simulink model "DFIG_BESS_In_power_LFnetwork_5bus"  (R2017b)
settings: Solver=ode23tb  StartTime=0.0  StopTime=7.5  MaxStep=0.04  RelTol=1e-3  EnableMultiTasking=on
undefined symbols (not defined in the file or in its folder): beta, Cbus, Cbus_bess, Cfilter, cp_opt_abs, D, D1, D11, Delta, DiscIntNeverNeededParam, f, Fs, fsw, Ion, J, ki_id, ki_idg, ki_iq, ki_iqg, ki_v, kp_id, kp_idg, kp_iq, kp_iqg, kp_v, Kpg, Kqg, lambda_opt, Lfilter, Lg, Lithium, Lm, Lr, Ls, Lsi, n, N, p, Ps, Radio, Rfilter, ro, Rr, Rs, sigbuilder_block, sigma, Ts, Vbus_ref, Vdc_bat_ref, Vs
libraries: powerlib x83, powerlib_meascontrol x28, sps_avr x2, electricdrivelib x1, peGeneralControl x1
(part 3 of 3)

== system DFIG_BESS_In_power_LFnetwork_5bus/BESS 1.0 MW 690 V/Control System/Charging Control ==
  "Pot_ref " : Inport
  "Pot_means " : Inport  Port=2
  Discrete-Time Integrator1 : DiscreteIntegrator  gainval=1  SampleTime=1/fsw  LimitOutput=on  UpperSaturationLimit=1200  LowerSaturationLimit=-1200  ICPrevOutput=DiscIntNeverNeededParam  ICPrevScaledInput=DiscIntNeverNeededParam
  Display6 : Display
  Error : Display
  Gain1 : Gain  Gain=Kpg
  Gain4 : Gain  Gain=Kpg*0.25
  Gain5 : Gain  Gain=0.03
  Mean : Display
  Mux : Mux  Inputs=3
  Ref : Display
  Sat : Display
  Sat1 : Display
  Saturation : Saturate  UpperLimit=1200  LowerLimit=-1200
  Scope : Scope
  Sum2 : Sum  Inputs=|+-
  Sum3 : Sum  Inputs=|++
  Id*_P : Outport
  wires:
  Sum2/1 -> Error/1, Mux/3, Gain5/1, Gain4/1
  Gain1/1 -> Display6/1
  Gain4/1 -> Sum3/1
  Sum3/1 -> Saturation/1
  Gain5/1 -> Discrete-Time Integrator1/1
  Discrete-Time Integrator1/1 -> Sat1/1, Sum3/2
  Mux/1 -> Scope/1
  "Pot_ref "/1 -> Mux/1, Ref/1, Gain1/1, Sum2/1
  "Pot_means "/1 -> Mux/2, Mean/1, Sum2/2
  Saturation/1 -> Sat/1, Id*_P/1

== system DFIG_BESS_In_power_LFnetwork_5bus/BESS 1.0 MW 690 V/Control System/Decoupling Idq ==
  Vd : Inport
  Vq : Inport  Port=2
  Fcn : Fcn  Expr=u[1]-u[4]*Lfilter*(2*pi*f)
  Fcn1 : Fcn  Expr=u[2]+u[3]*Lfilter*(2*pi*f)
  Mux1 : Mux
  Sum : Sum  Inputs=|++
  Sum1 : Sum  Inputs=|++
  " Vd_bat_ref" : Outport
  " Vq_bat_ref" : Outport  Port=2
  tag scope: Vd=global, Vq=global
  wires:
  Vd/1 -> Mux1/1
  Vq/1 -> Mux1/2
  Mux1/1 -> Fcn1/1, Fcn/1
  [id_bess] -> Mux1/3
  [iq_bess] -> Mux1/4
  Sum1/1 -> [Vq], " Vq_bat_ref"/1
  Fcn1/1 -> Sum1/1  "Vq*"
  Fcn/1 -> Sum/1  "Vd*"
  Sum/1 -> [Vd], " Vd_bat_ref"/1
  [Vd_bess] -> Sum/2
  [Vq_bess] -> Sum1/2

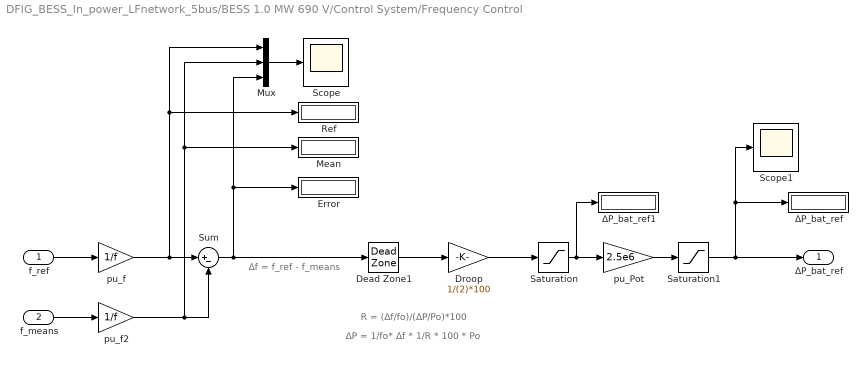
== system DFIG_BESS_In_power_LFnetwork_5bus/BESS 1.0 MW 690 V/Control System/Frequency Control ==
  note: Δf = f_ref - f_means
  note: R = (Δf/fo)/(ΔP/Po)*100
  note: ΔP = 1/fo* Δf * 1/R * 100 * Po
  f_ref : Inport
  f_means : Inport  Port=2
  Dead Zone1 : DeadZone  LowerValue=-0.00012*1/f  UpperValue=0.00002*1/f  SaturateOnIntegerOverflow=on
  Droop : Gain  Gain=1/(2)*100
  Error : Display
  Mean : Display
  Mux : Mux  Inputs=3
  Ref : Display
  Saturation : Saturate  UpperLimit=1  LowerLimit=0
  Saturation1 : Saturate  UpperLimit=1.5e6  LowerLimit=0
  Scope : Scope
  Scope1 : Scope
  Sum : Sum  Inputs=|+-
  "pu_Pot " : Gain  Gain=2.5e6
  pu_f : Gain  Gain=1/f
  pu_f2 : Gain  Gain=1/f
  ΔP_bat_ref : Display
  ΔP_bat_ref1 : Display
  "ΔP_bat_ref " : Outport
  wires:
  Mux/1 -> Scope/1
  f_ref/1 -> pu_f/1
  f_means/1 -> pu_f2/1
  Droop/1 -> Saturation/1
  Sum/1 -> Dead Zone1/1, Mux/3, Error/1
  Saturation/1 -> ΔP_bat_ref1/1, "pu_Pot "/1
  pu_f/1 -> Sum/1, Mux/1, Ref/1
  pu_f2/1 -> Sum/2, Mux/2, Mean/1
  "pu_Pot "/1 -> Saturation1/1
  Saturation1/1 -> Scope1/1, ΔP_bat_ref/1, "ΔP_bat_ref "/1
  Dead Zone1/1 -> Droop/1

== system DFIG_BESS_In_power_LFnetwork_5bus/BESS 1.0 MW 690 V/Control System/I* ==
  Id* : Inport
  Iq* : Inport  Port=2
  Display28 : Display
  Fcn : Fcn  Expr=sqrt((u[1])^2+(u[2])^2)
  Mux1 : Mux  Inputs=2
  "I* " : Outport
  wires:
  Fcn/1 -> Display28/1, "I* "/1
  Mux1/1 -> Fcn/1
  Id*/1 -> Mux1/1
  Iq*/1 -> Mux1/2

== system DFIG_BESS_In_power_LFnetwork_5bus/BESS 1.0 MW 690 V/Control System/Imean ==
  Id* : Inport
  Iq* : Inport  Port=2
  Display28 : Display
  Fcn : Fcn  Expr=sqrt((u[1])^2+(u[2])^2)
  Mux1 : Mux  Inputs=2
  "I* " : Outport
  wires:
  Iq*/1 -> Mux1/2
  Id*/1 -> Mux1/1
  Mux1/1 -> Fcn/1
  Fcn/1 -> Display28/1, "I* "/1

== system DFIG_BESS_In_power_LFnetwork_5bus/BESS 1.0 MW 690 V/Control System/P Control ==
  "Pot_ref " : Inport
  "Pot_means " : Inport  Port=2
  Discrete-Time Integrator1 : DiscreteIntegrator  gainval=1  SampleTime=1/fsw  LimitOutput=on  UpperSaturationLimit=3.5e6  LowerSaturationLimit=-1.5e6  ICPrevOutput=DiscIntNeverNeededParam  ICPrevScaledInput=DiscIntNeverNeededParam
  Error : Display
  Gain5 : Gain  Gain=Kpg
  Gain6 : Gain  Gain=kp_idg*1.1
  Gain7 : Gain  Gain=ki_idg*2.5
  Mean : Display
  Mux : Mux  Inputs=3
  Ref : Display
  Sat : Display
  Sat1 : Display
  Sat2 : Display
  Saturation : Saturate  UpperLimit=3.5e6  LowerLimit=-1.5e6
  Scope : Scope
  Sum2 : Sum  Inputs=|+-
  Sum3 : Sum  Inputs=|++
  Id*_P : Outport
  wires:
  Sum2/1 -> Error/1, Mux/3, Gain6/1, Gain7/1
  Gain6/1 -> Sum3/1, Sat2/1
  Sum3/1 -> Saturation/1
  Gain7/1 -> Discrete-Time Integrator1/1
  Discrete-Time Integrator1/1 -> Sat1/1, Sum3/2
  Mux/1 -> Scope/1
  "Pot_ref "/1 -> Sum2/1, Mux/1, Ref/1
  "Pot_means "/1 -> Mux/2, Mean/1, Sum2/2
  Saturation/1 -> Gain5/1, Sat/1
  Gain5/1 -> Id*_P/1

== system DFIG_BESS_In_power_LFnetwork_5bus/BESS 1.0 MW 690 V/Control System/PI Id1 ==
  idg_ref : Inport
  idg_means : Inport  Port=2
  Discrete-Time Integrator : DiscreteIntegrator  SampleTime=1/fsw  LimitOutput=on  UpperSaturationLimit=Vbus_ref/sqrt(3)*7  LowerSaturationLimit=-Vbus_ref/sqrt(3)*7  ICPrevOutput=DiscIntNeverNeededParam  ICPrevScaledInput=DiscIntNeverNeededParam
  Error : Display
  Gain : Gain  Gain=kp_idg
  Gain1 : Gain  Gain=ki_idg
  Mean : Display
  Mux : Mux  Inputs=3
  Ref : Display
  Sat : Display
  Sat 1 : Display
  Saturation : Saturate  UpperLimit=Vbus_ref/sqrt(3)*7  LowerLimit=-Vbus_ref/sqrt(3)*7
  Scope : Scope
  Sum : Sum  Inputs=|+-
  Sum1 : Sum  Inputs=|++
  out : Outport
  wires:
  Saturation/1 -> Sat/1, out/1
  Sum1/1 -> Saturation/1
  Discrete-Time Integrator/1 -> Sat 1/1, Sum1/2
  Gain1/1 -> Discrete-Time Integrator/1
  Gain/1 -> Sum1/1
  idg_means/1 -> Mean/1, Mux/2, Sum/2
  idg_ref/1 -> Ref/1, Mux/1, Sum/1
  Sum/1 -> Gain/1, Gain1/1, Mux/3, Error/1
  Mux/1 -> Scope/1

== system DFIG_BESS_In_power_LFnetwork_5bus/BESS 1.0 MW 690 V/Control System/PI Iq ==
  iq_bat_ref : Inport
  iq_bat_means : Inport  Port=2
  Discrete-Time Integrator : DiscreteIntegrator  SampleTime=1/fsw  LimitOutput=on  UpperSaturationLimit=Vbus_ref/sqrt(3)*5  LowerSaturationLimit=-Vbus_ref/sqrt(3)*5  ICPrevOutput=DiscIntNeverNeededParam  ICPrevScaledInput=DiscIntNeverNeededParam
  Error : Display
  Gain : Gain  Gain=kp_iqg
  Gain1 : Gain  Gain=ki_iqg
  Mean : Display
  Mux : Mux  Inputs=3
  Ref : Display
  Sat : Display
  Sat 1 : Display
  Saturation : Saturate  UpperLimit=Vbus_ref/sqrt(3)*6  LowerLimit=-Vbus_ref/sqrt(3)*6
  Scope : Scope
  Sum : Sum  Inputs=|+-
  Sum1 : Sum  Inputs=|++
  "out " : Outport
  wires:
  Mux/1 -> Scope/1
  Sum/1 -> Gain1/1, Gain/1, Error/1, Mux/3
  iq_bat_ref/1 -> Mux/1, Ref/1, Sum/1
  iq_bat_means/1 -> Mux/2, Mean/1, Sum/2
  Saturation/1 -> "out "/1, Sat/1
  Gain/1 -> Sum1/1
  Gain1/1 -> Discrete-Time Integrator/1
  Discrete-Time Integrator/1 -> Sum1/2, Sat 1/1
  Sum1/1 -> Saturation/1

== system DFIG_BESS_In_power_LFnetwork_5bus/BESS 1.0 MW 690 V/Control System/Q Control ==
  Q*_ref : Inport
  Q_means : Inport  Port=2
  Discrete-Time Integrator : DiscreteIntegrator  SampleTime=1/fsw  LimitOutput=on  UpperSaturationLimit=1.5e6  LowerSaturationLimit=-1.5e6  ICPrevOutput=DiscIntNeverNeededParam  ICPrevScaledInput=DiscIntNeverNeededParam
  Error : Display
  Gain1 : Gain  Gain=kp_iqg*0.25
  Gain4 : Gain  Gain=ki_iqg
  Gain5 : Gain  Gain=Kqg
  Mean : Display
  Mux : Mux  Inputs=3
  Ref : Display
  Sat : Display
  Sat 1 : Display
  Sat1 : Display
  Saturation : Saturate  UpperLimit=1.5e6  LowerLimit=-1.5e6
  Scope : Scope
  Sum : Sum  Inputs=|+-
  Sum1 : Sum  Inputs=|++
  "Q " : Outport
  wires:
  Mux/1 -> Scope/1
  Sum/1 -> Gain4/1, Gain1/1, Error/1, Mux/3
  Q*_ref/1 -> Mux/1, Ref/1, Sum/1
  Q_means/1 -> Mux/2, Mean/1, Sum/2
  Gain1/1 -> Sat1/1, Sum1/1
  Gain4/1 -> Discrete-Time Integrator/1
  Discrete-Time Integrator/1 -> Sum1/2, Sat 1/1
  Sum1/1 -> Saturation/1
  Gain5/1 -> "Q "/1
  Saturation/1 -> Gain5/1, Sat/1

== system DFIG_BESS_In_power_LFnetwork_5bus/BESS 1.0 MW 690 V/Control System/Q Control2 ==
  V*_ref : Inport
  V_means : Inport  Port=2
  Discrete-Time Integrator : DiscreteIntegrator  SampleTime=1/fsw  LimitOutput=on  UpperSaturationLimit=1.5e6  LowerSaturationLimit=-1.5e6  ICPrevOutput=DiscIntNeverNeededParam  ICPrevScaledInput=DiscIntNeverNeededParam
  Error : Display
  Gain1 : Gain  Gain=kp_iqg*1e3
  Gain4 : Gain  Gain=ki_iqg*1e3
  Mean : Display
  Mux : Mux  Inputs=3
  Ref : Display
  Sat 1 : Display
  Sat2 : Display
  Saturation : Saturate  UpperLimit=1.5e6  LowerLimit=-1.5e6
  Scope : Scope
  Sum : Sum  Inputs=|+-
  Sum1 : Sum  Inputs=|++
  "V " : Outport
  wires:
  Sum/1 -> Error/1, Mux/3, Gain4/1, Gain1/1
  Mux/1 -> Scope/1
  V*_ref/1 -> Mux/1, Ref/1, Sum/1
  V_means/1 -> Mux/2, Mean/1, Sum/2
  Gain1/1 -> Sum1/1
  Gain4/1 -> Discrete-Time Integrator/1
  Discrete-Time Integrator/1 -> Sum1/2, Sat 1/1
  Sum1/1 -> Saturation/1
  Saturation/1 -> "V "/1, Sat2/1

== system DFIG_BESS_In_power_LFnetwork_5bus/BESS 1.0 MW 690 V/Control System/V* ==
  Vd* : Inport
  Vq* : Inport  Port=2
  Display28 : Display
  Fcn : Fcn  Expr=sqrt((u[1])^2+(u[2])^2)
  Mux1 : Mux  Inputs=2
  "V* " : Outport
  wires:
  Vq*/1 -> Mux1/2
  Vd*/1 -> Mux1/1
  Mux1/1 -> Fcn/1
  Fcn/1 -> "V* "/1, Display28/1

== system DFIG_BESS_In_power_LFnetwork_5bus/BESS 1.0 MW 690 V/Control System/Vbus Control ==
  note: signal
  note: reference
  "ref Vbus " : Inport
  "means Vbus " : Inport  Port=2
  Discrete-Time Integrator1 : DiscreteIntegrator  SampleTime=1/fsw  LimitOutput=on  UpperSaturationLimit=0.5e6  LowerSaturationLimit=-0.5e6  ICPrevOutput=DiscIntNeverNeededParam  ICPrevScaledInput=DiscIntNeverNeededParam
  Error : Display
  Gain2 : Gain  Gain=-1000
  Gain3 : Gain  Gain=-300000
  Mean : Display
  Mux : Mux  Inputs=3
  Ref : Display
  Sat : Display
  Sat 1 : Display
  Saturation1 : Saturate  UpperLimit=0.4e6  LowerLimit=-0.4e6
  Scope : Scope
  Sum2 : Sum  Inputs=|+-
  Sum3 : Sum  Inputs=|++
  P_SOC_ref : Outport
  wires:
  Discrete-Time Integrator1/1 -> Sat 1/1, Sum3/2
  Gain3/1 -> Discrete-Time Integrator1/1
  Sum3/1 -> Saturation1/1
  Gain2/1 -> Sum3/1
  Saturation1/1 -> Sat/1, P_SOC_ref/1
  "means Vbus "/1 -> Sum2/2, Mean/1, Mux/2
  "ref Vbus "/1 -> Sum2/1, Ref/1, Mux/1
  Sum2/1 -> Gain2/1, Gain3/1, Mux/3, Error/1
  Mux/1 -> Scope/1

== system DFIG_BESS_In_power_LFnetwork_5bus/BESS 1.0 MW 690 V/Control System/Vmean ==
  Vd* : Inport
  Vq* : Inport  Port=2
  Display28 : Display
  Fcn : Fcn  Expr=sqrt((u[1])^2+(u[2])^2)
  Mux1 : Mux  Inputs=2
  "V* " : Outport
  wires:
  Fcn/1 -> "V* "/1, Display28/1
  Mux1/1 -> Fcn/1
  Vd*/1 -> Mux1/1
  Vq*/1 -> Mux1/2

== system DFIG_BESS_In_power_LFnetwork_5bus/BESS 1.0 MW 690 V/Control System/abc - α//β   ==
  note: iβ_bat
  note: iα_bat
  iabc_bat : Inport
  Fcn : Fcn  Expr=2/3*(u[1]-u[2]/2-u[3]/2)
  Fcn1 : Fcn  Expr=2/3*(u[2]*(sqrt(3)/2)-u[3]*(sqrt(3)/2))
  Mux : Mux  Inputs=2
  i α/β_bat : Outport
  wires:
  Mux/1 -> i α/β_bat/1
  iabc_bat/1 -> Fcn1/1, Fcn/1
  Fcn/1 -> Mux/1
  Fcn1/1 -> Mux/2

== system DFIG_BESS_In_power_LFnetwork_5bus/BESS 1.0 MW 690 V/Control System/abc - α//β  1 ==
  note: iα_bat
  note: iβ_bat
  Vabc_bat : Inport
  Fcn : Fcn  Expr=2/3*(u[1]-u[2]/2-u[3]/2)
  Fcn1 : Fcn  Expr=2/3*(u[2]*(sqrt(3)/2)-u[3]*(sqrt(3)/2))
  Mux : Mux  Inputs=2
  V α/β_bat : Outport
  wires:
  Fcn1/1 -> Mux/2
  Fcn/1 -> Mux/1
  Vabc_bat/1 -> Fcn/1, Fcn1/1
  Mux/1 -> V α/β_bat/1

== system DFIG_BESS_In_power_LFnetwork_5bus/BESS 1.0 MW 690 V/Control System/abc - α//β  2 ==
  note: iβ_bat
  note: iα_bat
  iabc_bat : Inport
  Fcn : Fcn  Expr=2/3*(u[1]-u[2]/2-u[3]/2)
  Fcn1 : Fcn  Expr=2/3*(u[2]*(sqrt(3)/2)-u[3]*(sqrt(3)/2))
  Mux : Mux  Inputs=2
  i α/β_bat : Outport
  wires:
  Mux/1 -> i α/β_bat/1
  iabc_bat/1 -> Fcn1/1, Fcn/1
  Fcn/1 -> Mux/1
  Fcn1/1 -> Mux/2

== system DFIG_BESS_In_power_LFnetwork_5bus/BESS 1.0 MW 690 V/Control System/abc - α//β  3 ==
  note: iα_bat
  note: iβ_bat
  Vabc_bat : Inport
  Fcn : Fcn  Expr=2/3*(u[1]-u[2]/2-u[3]/2)
  Fcn1 : Fcn  Expr=2/3*(u[2]*(sqrt(3)/2)-u[3]*(sqrt(3)/2))
  Mux : Mux  Inputs=2
  V α/β_bat : Outport
  wires:
  Fcn1/1 -> Mux/2
  Fcn/1 -> Mux/1
  Vabc_bat/1 -> Fcn/1, Fcn1/1
  Mux/1 -> V α/β_bat/1

== system DFIG_BESS_In_power_LFnetwork_5bus/BESS 1.0 MW 690 V/Control System/d//q  α//β  ==
  Vdq_bat : Inport
  theta_bat (θ_bat) : Inport  Port=2
  Fcn : Fcn  Expr=u(1)*cos(u[3])-u[2]*sin(u[3])
  Fcn1 : Fcn  Expr=u(1)*sin(u[3])+u[2]*cos(u[3])
  Mux : Mux  Inputs=2
  Mux1 : Mux  Inputs=2
  "Vα/β_bat " : Outport
  wires:
  Mux/1 -> "Vα/β_bat "/1
  Fcn/1 -> Mux/1
  Fcn1/1 -> Mux/2
  Vdq_bat/1 -> Mux1/1
  theta_bat (θ_bat)/1 -> Mux1/2
  Mux1/1 -> Fcn/1, Fcn1/1

== system DFIG_BESS_In_power_LFnetwork_5bus/BESS 1.0 MW 690 V/Control System/α//β - abc ==
  V α/β_bat : Inport
  Fcn : Fcn  Expr=u(1)
  Fcn1 : Fcn  Expr=-(u[1]/2)+u[2]*(sqrt(3)/2)
  Fcn2 : Fcn  Expr=-(u[1]/2)-u[2]*(sqrt(3)/2)
  Mux : Mux  Inputs=3
  Vabc_bat : Outport
  wires:
  Mux/1 -> Vabc_bat/1
  V α/β_bat/1 -> Fcn2/1, Fcn1/1, Fcn/1
  Fcn/1 -> Mux/1
  Fcn1/1 -> Mux/2
  Fcn2/1 -> Mux/3

== system DFIG_BESS_In_power_LFnetwork_5bus/BESS 1.0 MW 690 V/Control System/α//β - d//q ==
  i α/β_bat : Inport
  theta_bat (θ_bat) : Inport  Port=2
  Fcn : Fcn  Expr=u(1)*cos(u[3])+u[2]*sin(u[3])
  Fcn1 : Fcn  Expr=-u(1)*sin(u[3])+u[2]*cos(u[3])
  Mux : Mux  Inputs=2
  Mux1 : Mux  Inputs=2
  i d/q_bat : Outport
  wires:
  Mux/1 -> i d/q_bat/1
  Fcn/1 -> Mux/1
  Fcn1/1 -> Mux/2
  i α/β_bat/1 -> Mux1/1
  theta_bat (θ_bat)/1 -> Mux1/2
  Mux1/1 -> Fcn1/1, Fcn/1

== system DFIG_BESS_In_power_LFnetwork_5bus/BESS 1.0 MW 690 V/Control System/α//β - d//q1 ==
  V α/β_bat : Inport
  theta_bat (θ_bat) : Inport  Port=2
  Fcn : Fcn  Expr=u(1)*cos(u[3])+u[2]*sin(u[3])
  Fcn1 : Fcn  Expr=-u(1)*sin(u[3])+u[2]*cos(u[3])
  Mux : Mux  Inputs=2
  Mux1 : Mux  Inputs=2
  V d/q_bat : Outport
  wires:
  Mux1/1 -> Fcn/1, Fcn1/1
  theta_bat (θ_bat)/1 -> Mux1/2
  V α/β_bat/1 -> Mux1/1
  Fcn1/1 -> Mux/2
  Fcn/1 -> Mux/1
  Mux/1 -> V d/q_bat/1

== system DFIG_BESS_In_power_LFnetwork_5bus/BESS 1.0 MW 690 V/Control System/α//β - d//q2 ==
  i α/β_bat : Inport
  theta_bat (θ_bat) : Inport  Port=2
  Fcn : Fcn  Expr=u(1)*cos(u[3])+u[2]*sin(u[3])
  Fcn1 : Fcn  Expr=-u(1)*sin(u[3])+u[2]*cos(u[3])
  Mux : Mux  Inputs=2
  Mux1 : Mux  Inputs=2
  i d/q_bat : Outport
  wires:
  Mux/1 -> i d/q_bat/1
  Fcn/1 -> Mux/1
  Fcn1/1 -> Mux/2
  i α/β_bat/1 -> Mux1/1
  theta_bat (θ_bat)/1 -> Mux1/2
  Mux1/1 -> Fcn1/1, Fcn/1

== system DFIG_BESS_In_power_LFnetwork_5bus/BESS 1.0 MW 690 V/Control System/α//β - d//q3 ==
  V α/β_bat : Inport
  theta_bat (θ_bat) : Inport  Port=2
  Fcn : Fcn  Expr=u(1)*cos(u[3])+u[2]*sin(u[3])
  Fcn1 : Fcn  Expr=-u(1)*sin(u[3])+u[2]*cos(u[3])
  Mux : Mux  Inputs=2
  Mux1 : Mux  Inputs=2
  V d/q_bat : Outport
  wires:
  Mux1/1 -> Fcn/1, Fcn1/1
  theta_bat (θ_bat)/1 -> Mux1/2
  V α/β_bat/1 -> Mux1/1
  Fcn1/1 -> Mux/2
  Fcn/1 -> Mux/1
  Mux/1 -> V d/q_bat/1

== system DFIG_BESS_In_power_LFnetwork_5bus/DFIG 2.0 MW 690 V1/Control/ Angle Rotor ==
  note: Theta_m (θm)
      | Electric
  note: theta_V θv
  note: The stator reference frame (α - β) is a stationary
      | reference frame.
  note: The relation between the mechanical angle of the shaft and the
      | electrical angle depends on the pole pairs of the machine:
      |
      | θm (electrical) = Pole * θm (mechanical)
  note: theta_s (θs)
  note: Vαs/βs
  note: θs=θv-90°
  note: θs=θr+θm
      | θr=θs-θm
  note: Vector control of the DFIM is performed in a synchronously rotating dq frame, in which the d-axis is aligned, in this case, with the stator flux space vector
  Theta_m (θm) Mechanic : Inport
  Vabcs : Inport  Port=2
  "Clarke: abc - αβ " : Subsystem
  Constant : Constant  Value=pi/2
  Demux : Demux  Outputs=2
  Manual Switch1 : ManualSwitch  CurrentSetting=0
  PLL (3ph)1 : powerlib_meascontrol/PLL/PLL (3ph)  Commented=on  Fmin=45  Par_Init=[0, 60]  ParK=[180, 3200, 1]  TcD=1e-4  MaxRateChangeFreq=12  FilterCutOffFreq=25  Ts=0  AGC=on
      link override Model/abc to dq0: Alignment=Aligned with phase A axis
  Pole Pairs : Gain  Gain=p
  Sum : Sum  Inputs=|+-
  Sum1 : Sum  Inputs=|+-
  θv=tan^(-1) (Vβ/Vα) : Trigonometry  Operator=atan2
  theta_r (θr) : Outport
  wires:
  Vabcs/1 -> PLL (3ph)1/1, "Clarke: abc - αβ "/1(Vabc)
  Demux/2 -> θv=tan^(-1) (Vβ/Vα)/1
  Demux/1 -> θv=tan^(-1) (Vβ/Vα)/2
  "Clarke: abc - αβ "/1("Vαs/βs ") -> Demux/1
  Constant/1 -> Sum/2
  Theta_m (θm) Mechanic/1 -> Pole Pairs/1
  Sum/1 -> Sum1/1
  Sum1/1 -> theta_r (θr)/1
  Pole Pairs/1 -> Sum1/2
  Manual Switch1/1 -> Sum/1
  θv=tan^(-1) (Vβ/Vα)/1 -> Manual Switch1/2
  PLL (3ph)1/2 -> Manual Switch1/1

== system DFIG_BESS_In_power_LFnetwork_5bus/DFIG 2.0 MW 690 V1/Control/3er Harmonic Inyection ==
  in : Inport
  Gain : Gain  Gain=-0.5
  MinMax : MinMax
  MinMax1 : MinMax  Function=max
  Scope : Scope
  Sum : Sum  Inputs=|++
  Sum1 : Sum  Inputs=|++
  out : Outport
  wires:
  in/1 -> Sum1/1, MinMax1/1, MinMax/1
  MinMax/1 -> Sum/1
  MinMax1/1 -> Sum/2
  Sum1/1 -> out/1
  Sum/1 -> Gain/1
  Gain/1 -> Scope/1, Sum1/2

== system DFIG_BESS_In_power_LFnetwork_5bus/DFIG 2.0 MW 690 V1/Control/Cancelation of cc ==
  note: Stator Flux
  note: Ωm rd/s
      | Mechanic
  note: ωs (Hz)
  note: Pole Pairs
  note: ωr = ωs - ωm
  note: ωs (rd/s)
  note: ωm (rd/s)
      | Electrical
  Vd : Inport
  Vq : Inport  Port=2
  omega_m (Ωm) : Inport  Port=3
  Constant : Constant  Value=f
  Constant1 : Constant  Value=Fs
  Fcn : Fcn  Expr=u[1]-u[5]*sigma*Lr*u[4]
  Fcn1 : Fcn  Expr=u[2]+u[5]*sigma*Lr*u[3]+u[5]*(Lm/Ls)*u[6]
  Gain : Gain  Gain=p
  Gain1 : Gain  Gain=2*pi
  Mux : Mux  Inputs=2
  Mux1 : Mux  Inputs=6
  Sum : Sum  Inputs=|+-
  Vdr  Vqr : Outport
  tag scope: omega_s=global, vdr=global, vqr=global
  wires:
  Mux/1 -> Vdr  Vqr/1
  Fcn/1 -> [vdr], Mux/1
  Fcn1/1 -> [vqr], Mux/2
  Vd/1 -> Mux1/1
  Vq/1 -> Mux1/2
  Mux1/1 -> Fcn1/1, Fcn/1
  [idr] -> Mux1/3
  [iqr] -> Mux1/4
  Constant1/1 -> Mux1/6
  omega_m (Ωm)/1 -> Gain/1
  Gain/1 -> Sum/2
  Constant/1 -> Gain1/1
  Gain1/1 -> [omega_s], Sum/1
  Sum/1 -> Mux1/5

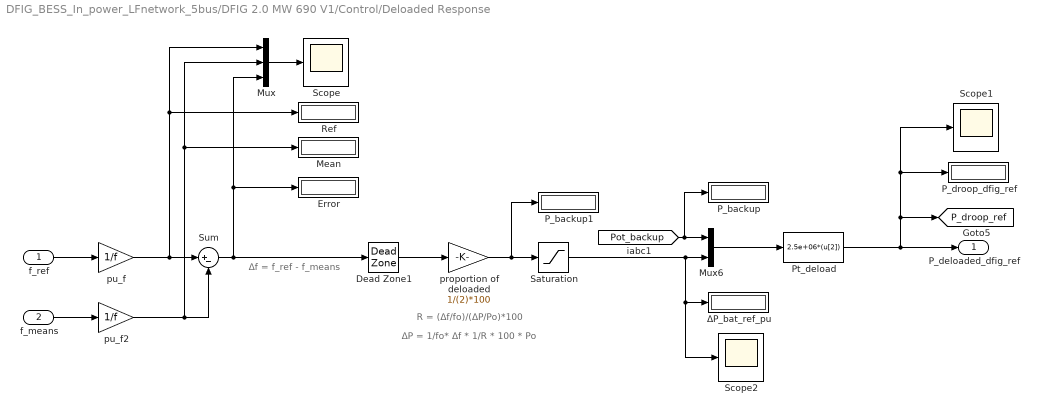
== system DFIG_BESS_In_power_LFnetwork_5bus/DFIG 2.0 MW 690 V1/Control/Deloaded Response ==
  note: Δf = f_ref - f_means
  note: R = (Δf/fo)/(ΔP/Po)*100
  note: ΔP = 1/fo* Δf * 1/R * 100 * Po
  f_ref : Inport
  f_means : Inport  Port=2
  Dead Zone1 : DeadZone  LowerValue=-0.00002*1/f  UpperValue=0.00002*1/f  SaturateOnIntegerOverflow=on
  Error : Display
  Mean : Display
  Mux : Mux  Inputs=3
  Mux6 : Mux  Inputs=2
  P_backup : Display
  P_backup1 : Display
  P_droop_dfig_ref : Display
  Pt_deload : Fcn  Expr=2.5e+06*(u[2])
  Ref : Display
  Saturation : Saturate  UpperLimit=1  LowerLimit=0
  Scope : Scope
  Scope1 : Scope
  Scope2 : Scope
  Sum : Sum  Inputs=|+-
  proportion of deloaded : Gain  Gain=1/(2)*100
  pu_f : Gain  Gain=1/f
  pu_f2 : Gain  Gain=1/f
  ΔP_bat_ref_pu : Display
  "P_deloaded_dfig_ref " : Outport
  tag scope: P_droop_ref=global
  wires:
  Mux/1 -> Scope/1
  f_ref/1 -> pu_f/1
  f_means/1 -> pu_f2/1
  proportion of deloaded/1 -> P_backup1/1, Saturation/1
  Sum/1 -> Dead Zone1/1, Mux/3, Error/1
  Saturation/1 -> Scope2/1, ΔP_bat_ref_pu/1, Mux6/2
  pu_f/1 -> Sum/1, Mux/1, Ref/1
  pu_f2/1 -> Sum/2, Mux/2, Mean/1
  Pt_deload/1 -> "P_deloaded_dfig_ref "/1, [P_droop_ref], Scope1/1, P_droop_dfig_ref/1
  Dead Zone1/1 -> proportion of deloaded/1
  Mux6/1 -> Pt_deload/1
  [Pot_backup] -> P_backup/1, Mux6/1

== system DFIG_BESS_In_power_LFnetwork_5bus/DFIG 2.0 MW 690 V1/Control/Inertial Response ==
  note: P = 2H*w*df/dt
  note: P = 1/2*(J*wo^2)/(Ps)
  f_means : Inport
  Filtered Derivative (Discrete or Continuous) : peGeneralControl/Filtered Derivative (Discrete or Continuous)  K=1  T=0.1  B=inf  A=-inf  minRatio=10  Ts=-1
  H: Inertia constant : Constant  Value=1/2*(J*(n*2*pi/60)^2)/(Ps)
  Inertial_Res : Fcn  Expr=2*u[1]*u[2]*u[3]
  Inertial_response : Display
  Mux1 : Mux  Inputs=3
  "P_pu -> P [W]1" : Gain  Gain=2.5e+06
  Scope1 : Scope
  display : Display
  display2 : Display
  f_pu : Gain  Gain=1/f
  w_pu1 : Gain  Gain=1/(n*2*pi/60)
  "Inertial_Res " : Outport
  tag scope: I_reponse_ref=global
  wires:
  [omega_m] -> w_pu1/1  "Rotor speed"
  H: Inertia constant/1 -> Mux1/1, display/1
  Mux1/1 -> Inertial_Res/1
  f_means/1 -> f_pu/1
  Filtered Derivative (Discrete or Continuous)/1 -> display2/1, Mux1/3
  f_pu/1 -> Filtered Derivative (Discrete or Continuous)/1
  Inertial_Res/1 -> "P_pu -> P [W]1"/1
  "P_pu -> P [W]1"/1 -> [I_reponse_ref], Scope1/1, Inertial_response/1, "Inertial_Res "/1
  w_pu1/1 -> Mux1/2

== system DFIG_BESS_In_power_LFnetwork_5bus/DFIG 2.0 MW 690 V1/Control/Inertial Response1 ==
  note: Is f > 59.96? ONS Brazil
  note: Yes
  note: No
  f_means : Inport
  P_deloaded : Inport  Port=2
  P_max : Inport  Port=3
  P_deloaded_ref : Display
  P_deloaded_ref1 : Display
  P_deloaded_ref2 : Display
  SOC / POWER Switch1 : Switch  Criteria=u2 > Threshold  Threshold=59.97
  Scope2 : Scope
  "P_deloaded " : Outport
  tag scope: P_reserve_ref=global
  wires:
  f_means/1 -> SOC / POWER Switch1/2
  P_deloaded/1 -> P_deloaded_ref1/1, SOC / POWER Switch1/1
  SOC / POWER Switch1/1 -> Scope2/1, P_deloaded_ref/1, [P_reserve_ref], "P_deloaded "/1
  P_max/1 -> SOC / POWER Switch1/3, P_deloaded_ref2/1

== system DFIG_BESS_In_power_LFnetwork_5bus/DFIG 2.0 MW 690 V1/Control/P Control ==
  "Pot_ref " : Inport
  "Pot_means " : Inport  Port=2
  Discrete-Time Integrator1 : DiscreteIntegrator  gainval=1  SampleTime=1/fsw  LimitOutput=on  UpperSaturationLimit=3500  LowerSaturationLimit=-3500  ICPrevOutput=DiscIntNeverNeededParam  ICPrevScaledInput=DiscIntNeverNeededParam
  Error : Display
  Gain3 : Gain  Gain=kp_iq/1e2
  Gain4 : Gain  Gain=kp_iq/1e5
  Gain5 : Gain  Gain=ki_iq/1e+02
  Gain6 : Gain  Gain=ki_iq/1e4
  Mean : Display
  Mux : Mux  Inputs=3
  Ref : Display
  Sat : Display
  Sat1 : Display
  Sat2 : Display
  Scope : Scope
  Sum2 : Sum  Inputs=|+-
  Sum3 : Sum  Inputs=|++
  Id*_P : Outport
  wires:
  Gain5/1 -> Sum3/1, Sat2/1
  Gain4/1 -> Discrete-Time Integrator1/1
  Discrete-Time Integrator1/1 -> Sat1/1, Sum3/2
  Mux/1 -> Scope/1
  "Pot_ref "/1 -> Sum2/1, Ref/1, Mux/1
  "Pot_means "/1 -> Mux/2, Mean/1, Sum2/2
  Sum3/1 -> Sat/1, Id*_P/1
  Sum2/1 -> Error/1, Mux/3, Gain5/1, Gain4/1

== system DFIG_BESS_In_power_LFnetwork_5bus/DFIG 2.0 MW 690 V1/Control/P Control1 ==
  "T_ref " : Inport
  "T_means " : Inport  Port=2
  Discrete-Time Integrator1 : DiscreteIntegrator  gainval=1  SampleTime=1/fsw  LimitOutput=on  ICPrevOutput=DiscIntNeverNeededParam  ICPrevScaledInput=DiscIntNeverNeededParam
  Error : Display
  Gain1 : Gain  Gain=-1
  Gain5 : Gain  Gain=kp_iq/1e5
  Gain6 : Gain  Gain=ki_iq*1.5/1e2
  Mean : Display
  Mux : Mux  Inputs=3
  Ref : Display
  Sat : Display
  Sat1 : Display
  Sat2 : Display
  Scope : Scope
  Scope1 : Scope
  Sum2 : Sum  Inputs=|+-
  Sum3 : Sum  Inputs=|++
  Id*_P : Outport
  wires:
  Sum2/1 -> Gain5/1, Gain6/1, Mux/3, Error/1
  "T_means "/1 -> Sum2/2, Mean/1, Mux/2
  "T_ref "/1 -> Ref/1, Mux/1, Sum2/1
  Mux/1 -> Scope/1
  Discrete-Time Integrator1/1 -> Sum3/2, Sat1/1
  Gain5/1 -> Discrete-Time Integrator1/1
  Gain6/1 -> Sat2/1, Sum3/1
  Gain1/1 -> Id*_P/1, Scope1/1, Sat/1
  Sum3/1 -> Gain1/1

== system DFIG_BESS_In_power_LFnetwork_5bus/DFIG 2.0 MW 690 V1/Control/PI Id ==
  idr_ref : Inport
  idr_means : Inport  Port=2
  Discrete-Time Integrator : DiscreteIntegrator  SampleTime=1/fsw  LimitOutput=on  UpperSaturationLimit=Vbus_ref/sqrt(3)  LowerSaturationLimit=-Vbus_ref/sqrt(3)  ICPrevOutput=DiscIntNeverNeededParam  ICPrevScaledInput=DiscIntNeverNeededParam
  Error : Display
  Gain : Gain  Gain=kp_id
  Gain1 : Gain  Gain=ki_id
  Mean : Display
  Mux : Mux  Inputs=3
  Ref : Display
  Sat : Display
  Sat2 : Display
  Saturation : Saturate  UpperLimit=Vbus_ref/sqrt(3)  LowerLimit=-Vbus_ref/sqrt(3)
  Scope : Scope
  Sum : Sum  Inputs=|+-
  Sum1 : Sum  Inputs=|++
  Vd : Outport
  wires:
  idr_means/1 -> Mean/1, Mux/2, Sum/2
  idr_ref/1 -> Ref/1, Mux/1, Sum/1
  Sum/1 -> Gain/1, Gain1/1, Mux/3, Error/1
  Gain/1 -> Sum1/1
  Gain1/1 -> Discrete-Time Integrator/1
  Discrete-Time Integrator/1 -> Sat2/1, Sum1/2
  Sum1/1 -> Saturation/1
  Saturation/1 -> Sat/1, Vd/1
  Mux/1 -> Scope/1

== system DFIG_BESS_In_power_LFnetwork_5bus/DFIG 2.0 MW 690 V1/Control/PI Iq ==
  iqr_ref : Inport
  iqr_means : Inport  Port=2
  Discrete-Time Integrator : DiscreteIntegrator  SampleTime=1/fsw  LimitOutput=on  UpperSaturationLimit=Vbus_ref/sqrt(3)  LowerSaturationLimit=-Vbus_ref/sqrt(3)  ICPrevOutput=DiscIntNeverNeededParam  ICPrevScaledInput=DiscIntNeverNeededParam
  Display1 : Display
  Error : Display
  Gain : Gain  Gain=kp_iq
  Gain1 : Gain  Gain=ki_iq
  Mean : Display
  Mux : Mux  Inputs=3
  Ref : Display
  Sat : Display
  Saturation : Saturate  UpperLimit=Vbus_ref/sqrt(3)  LowerLimit=-Vbus_ref/sqrt(3)
  Scope : Scope
  Sum : Sum  Inputs=|+-
  Sum1 : Sum  Inputs=|++
  Vq : Outport
  wires:
  Gain/1 -> Sum1/1
  Gain1/1 -> Discrete-Time Integrator/1
  Sum1/1 -> Saturation/1
  Discrete-Time Integrator/1 -> Display1/1, Sum1/2
  iqr_means/1 -> Sum/2, Mean/1, Mux/2
  iqr_ref/1 -> Sum/1, Ref/1, Mux/1
  Sum/1 -> Gain/1, Gain1/1, Mux/3, Error/1
  Saturation/1 -> Sat/1, Vq/1
  Mux/1 -> Scope/1

== system DFIG_BESS_In_power_LFnetwork_5bus/DFIG 2.0 MW 690 V1/Control/abc - α//β  ==
  note: iβr
  note: iαr
  iabcr : Inport
  Fcn : Fcn  Expr=2/3*(u[1]-u[2]/2-u[3]/2)
  Fcn1 : Fcn  Expr=2/3*(u[2]*(sqrt(3)/2)-u[3]*(sqrt(3)/2))
  Mux : Mux  Inputs=2
  i αr/βr : Outport
  wires:
  Mux/1 -> i αr/βr/1
  iabcr/1 -> Fcn1/1, Fcn/1
  Fcn/1 -> Mux/1
  Fcn1/1 -> Mux/2

== system DFIG_BESS_In_power_LFnetwork_5bus/DFIG 2.0 MW 690 V1/Control/d//q - α//β ==
  Vdr  Vqr : Inport
  theta_r (θr) : Inport  Port=2
  Fcn : Fcn  Expr=u(1)*cos(u[3])-u[2]*sin(u[3])
  Fcn1 : Fcn  Expr=u(1)*sin(u[3])+u[2]*cos(u[3])
  Mux : Mux  Inputs=2
  Mux1 : Mux  Inputs=2
  V αr/βr : Outport
  wires:
  Mux/1 -> V αr/βr/1
  Fcn/1 -> Mux/1
  Fcn1/1 -> Mux/2
  Vdr  Vqr/1 -> Mux1/1
  theta_r (θr)/1 -> Mux1/2
  Mux1/1 -> Fcn/1, Fcn1/1

== system DFIG_BESS_In_power_LFnetwork_5bus/DFIG 2.0 MW 690 V1/Control/α//β - abc ==
  V αr/βr : Inport
  Fcn : Fcn  Expr=u(1)
  Fcn1 : Fcn  Expr=-(u[1]/2)+u[2]*(sqrt(3)/2)
  Fcn2 : Fcn  Expr=-(u[1]/2)-u[2]*(sqrt(3)/2)
  Mux : Mux  Inputs=3
  Vabcr : Outport
  wires:
  Mux/1 -> Vabcr/1
  V αr/βr/1 -> Fcn2/1, Fcn1/1, Fcn/1
  Fcn/1 -> Mux/1
  Fcn1/1 -> Mux/2
  Fcn2/1 -> Mux/3

== system DFIG_BESS_In_power_LFnetwork_5bus/DFIG 2.0 MW 690 V1/Control/α//β - d//q ==
  i αr/βr : Inport
  theta_r (θr) : Inport  Port=2
  Fcn : Fcn  Expr=u(1)*cos(u[3])+u[2]*sin(u[3])
  Fcn1 : Fcn  Expr=-u(1)*sin(u[3])+u[2]*cos(u[3])
  Mux : Mux  Inputs=2
  Mux1 : Mux  Inputs=2
  i dr/qr : Outport
  wires:
  Mux/1 -> i dr/qr/1
  Fcn/1 -> Mux/1
  Fcn1/1 -> Mux/2
  i αr/βr/1 -> Mux1/1
  theta_r (θr)/1 -> Mux1/2
  Mux1/1 -> Fcn1/1, Fcn/1

== system DFIG_BESS_In_power_LFnetwork_5bus/DFIG 2.0 MW 690 V1/Control1/ Angle Rotor ==
  note: Vg α/β
  "Vabcg " : Inport
  " abc - αβ " : Subsystem
  Demux : Demux  Outputs=2
  θv=tan^(-1) (Vβ/Vα) : Trigonometry  Operator=atan2
  theta_g (θg) : Outport
  wires:
  " abc - αβ "/1("Vg α/β ") -> Demux/1
  Demux/1 -> θv=tan^(-1) (Vβ/Vα)/2
  Demux/2 -> θv=tan^(-1) (Vβ/Vα)/1
  "Vabcg "/1 -> " abc - αβ "/1(Vabcg)
  θv=tan^(-1) (Vβ/Vα)/1 -> theta_g (θg)/1

== system DFIG_BESS_In_power_LFnetwork_5bus/DFIG 2.0 MW 690 V1/Control1/3er Harmonic Inyection ==
  in : Inport
  Gain : Gain  Gain=-0.5
  MinMax : MinMax
  MinMax1 : MinMax  Function=max
  Scope : Scope
  Sum : Sum  Inputs=|++
  Sum1 : Sum  Inputs=|++
  out : Outport
  wires:
  Gain/1 -> Sum1/2, Scope/1
  Sum/1 -> Gain/1
  Sum1/1 -> out/1
  MinMax1/1 -> Sum/2
  MinMax/1 -> Sum/1
  in/1 -> MinMax/1, MinMax1/1, Sum1/1

== system DFIG_BESS_In_power_LFnetwork_5bus/DFIG 2.0 MW 690 V1/Control1/Cancelation of cc ==
  Id : Inport
  Iq : Inport  Port=2
  Display : Display
  Fcn : Fcn  Expr=u[1]-u[4]*Lg*(2*pi*f)
  Fcn1 : Fcn  Expr=u[2]+u[3]*Lg*(2*pi*f)
  Mux : Mux  Inputs=2
  Mux1 : Mux
  Vdg  Vqg : Outport
  tag scope: vdg=global, vqg=global
  wires:
  [iqg] -> Mux1/4
  [idg] -> Mux1/3
  Mux1/1 -> Fcn/1, Fcn1/1
  Iq/1 -> Mux1/2
  Id/1 -> Mux1/1
  Fcn1/1 -> Mux/2, [vqg]
  Fcn/1 -> Mux/1, Display/1, [vdg]
  Mux/1 -> Vdg  Vqg/1

== system DFIG_BESS_In_power_LFnetwork_5bus/DFIG 2.0 MW 690 V1/Control1/PI ==
  note: signal
  note: reference
  "ref Vbus " : Inport
  "means Vbus " : Inport  Port=2
  Discrete-Time Integrator1 : DiscreteIntegrator  SampleTime=1/fsw  LimitOutput=on  UpperSaturationLimit=Ps  LowerSaturationLimit=-Ps  ICPrevOutput=DiscIntNeverNeededParam  ICPrevScaledInput=DiscIntNeverNeededParam
  Error : Display
  Gain2 : Gain  Gain=kp_v*80
  Gain3 : Gain  Gain=ki_v*0.9/1e+03
  Mean : Display
  Mux : Mux  Inputs=3
  Ref : Display
  Sat : Display
  Sat 1 : Display
  Sat1 : Display
  Saturation1 : Saturate  UpperLimit=Ps  LowerLimit=-Ps
  Scope : Scope
  Sum2 : Sum  Inputs=|+-
  Sum3 : Sum  Inputs=|++
  P_rotor_ref : Outport
  wires:
  Discrete-Time Integrator1/1 -> Sat 1/1, Sum3/2
  Gain3/1 -> Discrete-Time Integrator1/1
  Sum3/1 -> Saturation1/1
  Gain2/1 -> Sat1/1, Sum3/1
  Saturation1/1 -> Sat/1, P_rotor_ref/1
  "means Vbus "/1 -> Sum2/2, Mean/1, Mux/2
  "ref Vbus "/1 -> Sum2/1, Ref/1, Mux/1
  Sum2/1 -> Gain2/1, Gain3/1, Mux/3, Error/1
  Mux/1 -> Scope/1

== system DFIG_BESS_In_power_LFnetwork_5bus/DFIG 2.0 MW 690 V1/Control1/PI Id ==
  idg_ref : Inport
  idg_means : Inport  Port=2
  Discrete-Time Integrator : DiscreteIntegrator  SampleTime=1/fsw  LimitOutput=on  UpperSaturationLimit=Vbus_ref/sqrt(3)*2  LowerSaturationLimit=-Vbus_ref/sqrt(3)*2  ICPrevOutput=DiscIntNeverNeededParam  ICPrevScaledInput=DiscIntNeverNeededParam
  Error : Display
  Gain : Gain  Gain=kp_idg
  Gain1 : Gain  Gain=ki_idg
  Mean : Display
  Mux : Mux  Inputs=3
  Ref : Display
  Sat : Display
  Sat 1 : Display
  Saturation : Saturate  UpperLimit=Vbus_ref/sqrt(3)*2  LowerLimit=-Vbus_ref/sqrt(3)*2
  Scope : Scope
  Sum : Sum  Inputs=|+-
  Sum1 : Sum  Inputs=|++
  out : Outport
  wires:
  Saturation/1 -> Sat/1, out/1
  Sum1/1 -> Saturation/1
  Discrete-Time Integrator/1 -> Sat 1/1, Sum1/2
  Gain1/1 -> Discrete-Time Integrator/1
  Gain/1 -> Sum1/1
  idg_means/1 -> Mean/1, Mux/2, Sum/2
  idg_ref/1 -> Ref/1, Mux/1, Sum/1
  Sum/1 -> Gain/1, Gain1/1, Mux/3, Error/1
  Mux/1 -> Scope/1

== system DFIG_BESS_In_power_LFnetwork_5bus/DFIG 2.0 MW 690 V1/Control1/PI Iq ==
  iqg_ref : Inport
  iqg_means : Inport  Port=2
  Discrete-Time Integrator : DiscreteIntegrator  SampleTime=1/fsw  LimitOutput=on  UpperSaturationLimit=Vbus_ref/sqrt(3)  LowerSaturationLimit=-Vbus_ref/sqrt(3)  ICPrevOutput=DiscIntNeverNeededParam  ICPrevScaledInput=DiscIntNeverNeededParam
  Error : Display
  Gain : Gain  Gain=kp_iqg
  Gain1 : Gain  Gain=ki_iqg
  Mean : Display
  Mux : Mux  Inputs=3
  Ref : Display
  Sat : Display
  Sat 1 : Display
  Saturation : Saturate  UpperLimit=Vbus_ref/sqrt(3)  LowerLimit=-Vbus_ref/sqrt(3)
  Scope : Scope
  Sum : Sum  Inputs=|+-
  Sum1 : Sum  Inputs=|++
  out : Outport
  wires:
  Sum1/1 -> Saturation/1
  Discrete-Time Integrator/1 -> Sat 1/1, Sum1/2
  Gain1/1 -> Discrete-Time Integrator/1
  Gain/1 -> Sum1/1
  Saturation/1 -> Sat/1, out/1
  iqg_means/1 -> Sum/2, Mean/1, Mux/2
  iqg_ref/1 -> Sum/1, Ref/1, Mux/1
  Sum/1 -> Mux/3, Error/1, Gain/1, Gain1/1
  Mux/1 -> Scope/1

== system DFIG_BESS_In_power_LFnetwork_5bus/DFIG 2.0 MW 690 V1/Control1/abc - α//β   ==
  note: iαg
  note: iβg
  iabcg : Inport
  Fcn : Fcn  Expr=2/3*(u[1]-u[2]/2-u[3]/2)
  Fcn1 : Fcn  Expr=2/3*(u[2]*(sqrt(3)/2)-u[3]*(sqrt(3)/2))
  Mux : Mux  Inputs=2
  i αg/βg : Outport
  wires:
  Fcn1/1 -> Mux/2
  Fcn/1 -> Mux/1
  iabcg/1 -> Fcn/1, Fcn1/1
  Mux/1 -> i αg/βg/1

== system DFIG_BESS_In_power_LFnetwork_5bus/DFIG 2.0 MW 690 V1/Control1/d//q  α//β  ==
  Vdg  Vqg : Inport
  theta_g (θg) : Inport  Port=2
  Fcn : Fcn  Expr=u(1)*cos(u[3])-u[2]*sin(u[3])
  Fcn1 : Fcn  Expr=u(1)*sin(u[3])+u[2]*cos(u[3])
  Mux : Mux  Inputs=2
  Mux1 : Mux  Inputs=2
  V αg/βg : Outport
  wires:
  Mux1/1 -> Fcn1/1, Fcn/1
  theta_g (θg)/1 -> Mux1/2
  Vdg  Vqg/1 -> Mux1/1
  Fcn1/1 -> Mux/2
  Fcn/1 -> Mux/1
  Mux/1 -> V αg/βg/1

== system DFIG_BESS_In_power_LFnetwork_5bus/DFIG 2.0 MW 690 V1/Control1/α//β - abc ==
  V αg/βg : Inport
  Fcn : Fcn  Expr=u(1)
  Fcn1 : Fcn  Expr=-(u[1]/2)+u[2]*(sqrt(3)/2)
  Fcn2 : Fcn  Expr=-(u[1]/2)-u[2]*(sqrt(3)/2)
  Mux : Mux  Inputs=3
  Vabcg : Outport
  wires:
  Fcn2/1 -> Mux/3
  Fcn1/1 -> Mux/2
  Fcn/1 -> Mux/1
  V αg/βg/1 -> Fcn/1, Fcn1/1, Fcn2/1
  Mux/1 -> Vabcg/1

== system DFIG_BESS_In_power_LFnetwork_5bus/DFIG 2.0 MW 690 V1/Control1/α//β - d//q ==
  i αg/βg : Inport
  theta_g (θg) : Inport  Port=2
  Fcn : Fcn  Expr=u(1)*cos(u[3])+u[2]*sin(u[3])
  Fcn1 : Fcn  Expr=-u(1)*sin(u[3])+u[2]*cos(u[3])
  Mux : Mux  Inputs=2
  Mux1 : Mux  Inputs=2
  i dg/qg : Outport
  wires:
  Mux1/1 -> Fcn/1, Fcn1/1
  theta_g (θg)/1 -> Mux1/2
  i αg/βg/1 -> Mux1/1
  Fcn1/1 -> Mux/2
  Fcn/1 -> Mux/1
  Mux/1 -> i dg/qg/1

== system DFIG_BESS_In_power_LFnetwork_5bus/BESS 1.0 MW 690 V/Control System/ Angle Rotor/ abc - αβ  ==
  Vabc_bat : Inport
  Fcn : Fcn  Expr=2/3*(u[1]-u[2]/2-u[3]/2)
  Fcn1 : Fcn  Expr=2/3*(u[2]*(sqrt(3)/2)-u[3]*(sqrt(3)/2))
  Mux : Mux  Inputs=2
  "V α/β_bat " : Outport
  wires:
  Mux/1 -> "V α/β_bat "/1
  Vabc_bat/1 -> Fcn1/1, Fcn/1
  Fcn/1 -> Mux/1
  Fcn1/1 -> Mux/2

== system DFIG_BESS_In_power_LFnetwork_5bus/BESS 1.0 MW 690 V/Control System/ Angle Rotor1/ abc - αβ  ==
  Vabc_bat : Inport
  Fcn : Fcn  Expr=2/3*(u[1]-u[2]/2-u[3]/2)
  Fcn1 : Fcn  Expr=2/3*(u[2]*(sqrt(3)/2)-u[3]*(sqrt(3)/2))
  Mux : Mux  Inputs=2
  "V α/β_bat " : Outport
  wires:
  Mux/1 -> "V α/β_bat "/1
  Vabc_bat/1 -> Fcn1/1, Fcn/1
  Fcn/1 -> Mux/1
  Fcn1/1 -> Mux/2

== system DFIG_BESS_In_power_LFnetwork_5bus/DFIG 2.0 MW 690 V1/Control/ Angle Rotor/Clarke: abc - αβ  ==
  Vabc : Inport
  Fcn : Fcn  Expr=2/3*(u[1]-u[2]/2-u[3]/2)
  Fcn1 : Fcn  Expr=2/3*(u[2]*(sqrt(3)/2)-u[3]*(sqrt(3)/2))
  Mux : Mux  Inputs=2
  "Vαs/βs " : Outport
  wires:
  Mux/1 -> "Vαs/βs "/1
  Vabc/1 -> Fcn1/1, Fcn/1
  Fcn/1 -> Mux/1
  Fcn1/1 -> Mux/2

== system DFIG_BESS_In_power_LFnetwork_5bus/DFIG 2.0 MW 690 V1/Control1/ Angle Rotor/ abc - αβ  ==
  Vabcg : Inport
  Fcn : Fcn  Expr=2/3*(u[1]-u[2]/2-u[3]/2)
  Fcn1 : Fcn  Expr=2/3*(u[2]*(sqrt(3)/2)-u[3]*(sqrt(3)/2))
  Mux : Mux  Inputs=2
  "Vg α/β " : Outport
  wires:
  Fcn1/1 -> Mux/2
  Fcn/1 -> Mux/1
  Vabcg/1 -> Fcn/1, Fcn1/1
  Mux/1 -> "Vg α/β "/1
